simulink model "combfilter"  (Simulink 6.0)
settings: Solver=FixedStepDiscrete  SolverMode=SingleTasking  StartTime=0.0  StopTime=4  RelTol=1e-3
settings Model: Creator=The MathWorks Inc.  LastModifiedBy=batserve  ExtModeTrigMode=oneshot  ExtModeArmWhenConnect=off  ExtModeAutoUpdateStatusClock=off
settings DataIOCC: LimitDataPoints=off  SaveFormat=Structure
settings OptimizationCC: BooleanDataType=off
settings DebuggingCC: CheckExecutionContextPreStartOutputMsg=on  CheckExecutionContextRuntimeOutputMsg=on  SolverPrmCheckMsg=none
settings HardwareCC: TargetUnknown=on

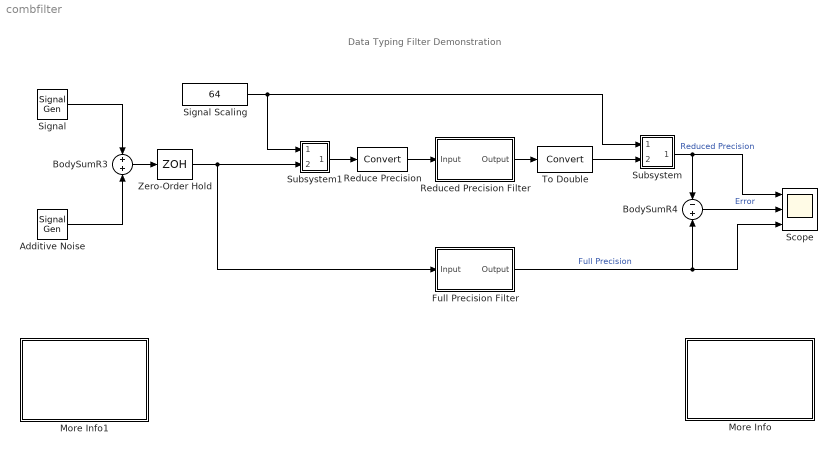
== system combfilter ==
  note: Data Typing Filter Demonstration
  Additive Noise : SignalGenerator  Amplitude=3  Frequency=25
      settings: AttributesFormatString=Waveform: %<Waveform>\nAmplitude: %<Amplitude>\nFreq: %<Frequency> %<Units>
  BodySumR3 : Sum  SaturateOnIntegerOverflow=on  InputSameDT=on
  BodySumR4 : Sum  Inputs=-+  SaturateOnIntegerOverflow=on  InputSameDT=on
  Full Precision Filter : Subsystem  PropExecContextAcrossSSBoundary=on
  More Info : Subsystem  PropExecContextAcrossSSBoundary=on
      mask Display: disp('Double click\nhere for\ninformation on\nthis demonstration')
  More Info1 : Subsystem  PropExecContextAcrossSSBoundary=on
      settings: OpenFcn=simcad(bdroot);
      mask Display: disp('Double click\nhere for\nSimulink Help')
  Reduce Precision : DataTypeConversion  OutDataTypeMode=single  SaturateOnIntegerOverflow=on  RndMeth=Zero
  Reduced Precision Filter : Subsystem  PropExecContextAcrossSSBoundary=on
  Scope : Scope  NumInputPorts=3
      settings: TimeRange=4  YMin=-400~-0.2~-400  YMax=400~0.2~400  DataFormat=Array
  Signal : SignalGenerator  Amplitude=100
      settings: AttributesFormatString=Waveform: %<Waveform>\nAmplitude: %<Amplitude>\nFreq: %<Frequency> %<Units>
  Signal Scaling : Constant  Value=64
  Subsystem : Subsystem  PropExecContextAcrossSSBoundary=on
      mask Display:
      | port_label('input',1,'/')
      | port_label('input',2,'x')
  Subsystem1 : Subsystem  PropExecContextAcrossSSBoundary=on
      mask Display: disp('X')
  To Double : DataTypeConversion  OutDataTypeMode=double  SaturateOnIntegerOverflow=on  RndMeth=Zero
  Zero-Order Hold : ZeroOrderHold  SampleTime=0.01
  wires:
  Reduced Precision Filter/1(Output) -> To Double/1
  Subsystem1/1(Out1) -> Reduce Precision/1
  To Double/1 -> Subsystem/2(In2)
  Zero-Order Hold/1 -> Subsystem1/2(In2), Full Precision Filter/1(Input)
  Subsystem/1(Out1) -> Scope/1, BodySumR4/1  "Reduced Precision"
  Reduce Precision/1 -> Reduced Precision Filter/1(Input)
  Signal Scaling/1 -> Subsystem/1(In1), Subsystem1/1(In1)
  Signal/1 -> BodySumR3/1
  Additive Noise/1 -> BodySumR3/2
  BodySumR3/1 -> Zero-Order Hold/1
  BodySumR4/1 -> Scope/2  "Error"
  Full Precision Filter/1(Output) -> Scope/3, BodySumR4/2  "Full Precision"

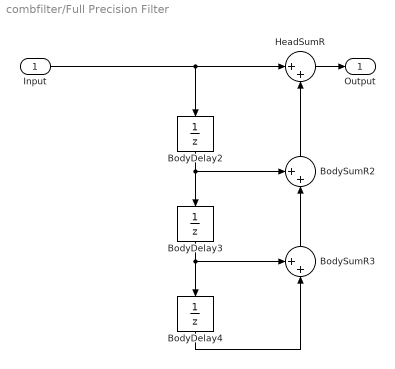
== system combfilter/Full Precision Filter ==
  Input : Inport  Port=1  LatchInput=off
  BodyDelay2 : UnitDelay  Orientation=down  SampleTime=-1
  BodyDelay3 : UnitDelay  Orientation=down  SampleTime=-1
  BodyDelay4 : UnitDelay  Orientation=down  SampleTime=-1
  BodySumR2 : Sum  Orientation=up  Inputs=++|  SaturateOnIntegerOverflow=on  InputSameDT=on
  BodySumR3 : Sum  Orientation=up  Inputs=++|  SaturateOnIntegerOverflow=on  InputSameDT=on
  HeadSumR : Sum  Inputs=|++  SaturateOnIntegerOverflow=on  InputSameDT=on
  Output : Outport
  wires:
  Input/1 -> BodyDelay2/1, HeadSumR/1
  BodyDelay2/1 -> BodyDelay3/1, BodySumR2/1
  BodyDelay3/1 -> BodyDelay4/1, BodySumR3/1
  BodyDelay4/1 -> BodySumR3/2
  BodySumR2/1 -> HeadSumR/2
  BodySumR3/1 -> BodySumR2/2
  HeadSumR/1 -> Output/1

== system combfilter/More Info ==
  note: Data Typing Filter Demonstration
  note: This demonstration shows how a filter can be applied to signals of different data types using
      | standard Simulink blocks.  In this example, a signal with some noise on it is produced.  This
      | signal is then fed into a filter as a single precision data type and a standard double data type.
      | The output from the filter for each signal is then compared and the error is displayed on the
      | scope.

== system combfilter/More Info1 ==

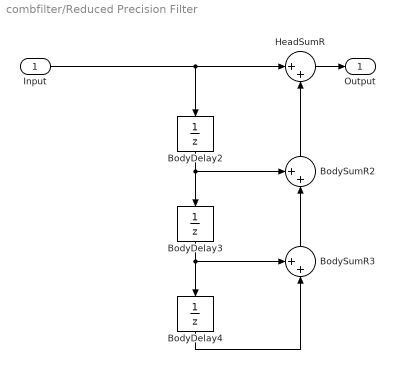
== system combfilter/Reduced Precision Filter ==
  Input : Inport  Port=1  LatchInput=off
  BodyDelay2 : UnitDelay  Orientation=down  SampleTime=-1
  BodyDelay3 : UnitDelay  Orientation=down  SampleTime=-1
  BodyDelay4 : UnitDelay  Orientation=down  SampleTime=-1
  BodySumR2 : Sum  Orientation=up  Inputs=++|  SaturateOnIntegerOverflow=on  InputSameDT=on
  BodySumR3 : Sum  Orientation=up  Inputs=++|  SaturateOnIntegerOverflow=on  InputSameDT=on
  HeadSumR : Sum  Inputs=|++  SaturateOnIntegerOverflow=on  InputSameDT=on
  Output : Outport
  wires:
  HeadSumR/1 -> Output/1
  BodySumR3/1 -> BodySumR2/2
  BodySumR2/1 -> HeadSumR/2
  BodyDelay4/1 -> BodySumR3/2
  BodyDelay3/1 -> BodySumR3/1, BodyDelay4/1
  BodyDelay2/1 -> BodySumR2/1, BodyDelay3/1
  Input/1 -> HeadSumR/1, BodyDelay2/1

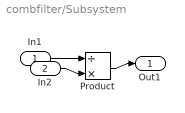
== system combfilter/Subsystem ==
  In1 : Inport  Port=1  LatchInput=off
  In2 : Inport  Port=2  LatchInput=off
  Product : Product  Inputs=/*  SaturateOnIntegerOverflow=on  RndMeth=Zero  InputSameDT=on
  Out1 : Outport
  wires:
  In1/1 -> Product/1
  Product/1 -> Out1/1
  In2/1 -> Product/2

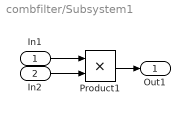
== system combfilter/Subsystem1 ==
  In1 : Inport  Port=1  LatchInput=off
  In2 : Inport  Port=2  LatchInput=off
  Product1 : Product  SaturateOnIntegerOverflow=on  RndMeth=Zero  InputSameDT=on
  Out1 : Outport
  wires:
  In2/1 -> Product1/2
  In1/1 -> Product1/1
  Product1/1 -> Out1/1
